simulink model "KalmanFilter_Testing"  (R2018a)
settings: Solver=VariableStepAuto  StartTime=0.0  StopTime=30  RelTol=1e-3
undefined symbols (not defined in the file): Continuous, d, dw, I, Iw, L, md, R, sampleTime, Time
libraries: simulink x2, cstblocks x2, ctrlSharedLib x1
settings Model: Creator=shravan  LastModifiedBy=shravan

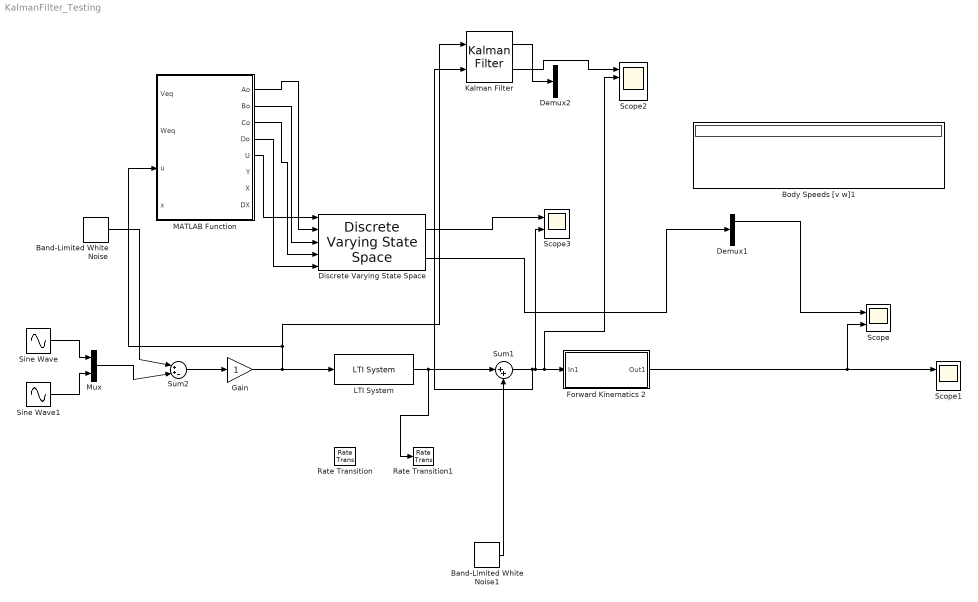
== system KalmanFilter_Testing ==
  Band-Limited White Noise : simulink/Sources/Band-Limited White Noise  Cov=0.001*sampleTime  Ts=sampleTime  seed=[23341]
  Band-Limited White Noise1 : simulink/Sources/Band-Limited White Noise  Cov=0.0001*sampleTime  Ts=sampleTime  seed=[23341]
  Body Speeds [v w]1 : Display
  Demux1 : Demux  Outputs=2
  Demux2 : Demux
  Discrete Varying State Space : cstblocks/Linear Parameter Varying/Discrete Varying State Space  x0=0  Ts=sampleTime  OutputX=on  OutputDX=off
      settings: SourceProductName=Control System Toolbox  SourceProductBaseCode=CT
  Forward Kinematics 2 : Subsystem
  Gain : Gain
  Kalman Filter : ctrlSharedLib/Kalman Filter  TimeDomain=Continuous-Time  UseCurrentEstimator=on  ModelSource=LTI State-Space Variable  ModelSourceVariable=Plant  A=0.95  B=1  C=1  D=0  NumberOfStates=1  NumberOfInputs=1  NumberOfOutputs=1  InitialEstimateSource=Dialog  X0=0  P0=10  UseK=off  UseGH=off  NumberOfProcessNoiseInputs=1  G=1  TimeInvariantG=on  H=0  TimeInvariantH=on  Q=0.05  TimeInvariantQ=on  R=1  TimeInvariantR=on  N=0  TimeInvariantN=on  AddInputPort=on  AddEnablePort=off  OutputEstimatedY=on  OutputP=off  Ts=-1
      settings: SourceProductBaseCode=CT
  LTI System : cstblocks/LTI System  sys=Plant  IC=[0 0 0 0]
  MATLAB Function : MATLAB Function  TreatAsAtomicUnit=on  SystemSampleTime=sampleTime
  Mux : Mux  Inputs=2
  Rate Transition : RateTransition  OutPortSampleTime=sampleTime
  Rate Transition1 : RateTransition  OutPortSampleTime=sampleTime
  Scope : Scope  NumInputPorts=2
  Scope1 : Scope  NumInputPorts=2
  Scope2 : Scope  NumInputPorts=4
  Scope3 : Scope  NumInputPorts=2
  Sine Wave : Sin  Bias=1
  Sine Wave1 : Sin  Bias=1  Phase=pi/4
  Sum1 : Sum  Inputs=|++
  Sum2 : Sum  Inputs=|++-
  wires:
  Gain/1 -> MATLAB Function/3(u), Kalman Filter/1, LTI System/1
  Kalman Filter/1 -> Demux2/1
  Sine Wave/1 -> Mux/1
  Sine Wave1/1 -> Mux/2
  Sum2/1 -> Gain/1
  Forward Kinematics 2/1(Out1) -> Scope/2, Scope1/1
  Band-Limited White Noise/1 -> Sum2/1
  Mux/1 -> Sum2/2
  Band-Limited White Noise1/1 -> Sum1/2
  Sum1/1 -> Kalman Filter/2, Scope3/2, Scope2/2, Forward Kinematics 2/1(In1)
  LTI System/1 -> Rate Transition1/1, Sum1/1
  MATLAB Function/1(Ao) -> Discrete Varying State Space/2
  MATLAB Function/2(Bo) -> Discrete Varying State Space/3
  MATLAB Function/3(Co) -> Discrete Varying State Space/4
  MATLAB Function/4(Do) -> Discrete Varying State Space/5
  Discrete Varying State Space/2 -> Demux1/1
  MATLAB Function/5(U) -> Discrete Varying State Space/1
  Discrete Varying State Space/1 -> Scope3/1
  Kalman Filter/2 -> Scope2/1
  Demux1/1 -> Scope/1

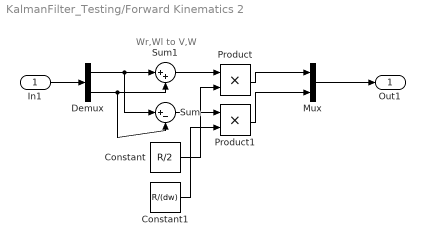
== system KalmanFilter_Testing/Forward Kinematics 2 ==
  note: Wr,Wl to V,W
  In1 : Inport
  Constant : Constant  Value=R/2
  Constant1 : Constant  Value=R/(dw)
  Demux : Demux  Outputs=2
  Mux : Mux  Inputs=2
  Product : Product
  Product1 : Product
  Sum : Sum  Inputs=|+-
  Sum1 : Sum  Inputs=|++
  Out1 : Outport
  wires:
  In1/1 -> Demux/1
  Product1/1 -> Mux/2
  Mux/1 -> Out1/1
  Product/1 -> Mux/1
  Demux/1 -> Sum/1, Sum1/1
  Demux/2 -> Sum/2, Sum1/2
  Sum1/1 -> Product/1
  Constant/1 -> Product/2
  Sum/1 -> Product1/1
  Constant1/1 -> Product1/2

== matlab function KalmanFilter_Testing/MATLAB Function ==
  data: Veq input size=[1,1]; Weq input size=[1,1]; u input size=[2,1]; Ao output size=[4,4]; x input size=[4,1]; Bo output size=[4,2]; Co output size=[2,4]; Do output size=[2,2]; U output size=[2,1]; Y output size=[2,1]; X output size=[4,1]; DX output size=[4,1]; sampleTime parameter size=[1,1]; d parameter size=[1,1]; dw parameter size=[1,1]; Iw parameter size=[1,1]; I parameter size=[1,1]; md parameter size=1,1; R parameter size=1,1; L parameter size=1,1
function [Ao,Bo,Co,Do,U,Y,X,DX] = fcn(Veq,Weq,u,x,sampleTime,d, dw, Iw, I, md, R, L)
% Sample time
Ts = sampleTime;
% Model Parameters
Kt = 0.0046; Kg = 50; Kb = Kt; Beta = 2.29e-06; La =1.729e-03; Ra = 5.51;
m = 3.4; mc = 2.76 + md; I = I ; Iw = Iw; L = L; d = d; dw = dw; 
A = m + 2*Iw/(R*R); B = I + dw*dw*Iw/(2*R*R);

% Continuous-time model for Plant e_r, e_l to Wr,Wl
Ac = [-2*Beta*Kg*Kg/(A*R*R)  2*mc*d*Weq/A   (Kt*Kg/(R*A))  (Kt*Kg/(A*R));
      -mc*d*Weq/B  (-mc*d*Veq/B)-(Beta*dw*dw*Kg*Kg/(2*R*R*B)) dw*Kt*Kg/(2*R*B) -dw*Kt*Kg/(2*B*R) ;
     -Kb*Kg/(La*R)   -Kb*Kg*dw/(2*La*R)  -Ra/La      0 ;
     -Kb*Kg/(La*R)    Kb*Kg*dw/(2*La*R)    0       -Ra/La ];
Bc = [0 0; 0 0; 1/La 0; 0 1/La]; Cc = [1/R dw/(2*R); 1/R -dw/(2*R)]*[1 0 0 0; 0 1 0 0]; Dc = [0 0;0 0];


% Discretize the continuous-time model using zero-order hold 
% on the inputs and a sample time of Ts seconds
nx = size(Ac,1);
nu = size(Bc,2);
M = expm([[Ac Bc]*Ts; zeros(nu,nx+nu)]);
Ao = M(1:nx,1:nx);
Bo = M(1:nx,nx+1:nx+nu);
Co = Cc;
Do = Dc;

% Nominal conditions for discrete-time plant
X = x;
U = u;
Y = Co*x + Do*u;
DX = Ao*x+Bo*u-x;
